simulink model "simulate"  (R2023a)
settings: Solver=VariableStepAuto  StartTime=0.0  StopTime=20  RelTol=1e-3
settings Model: Creator=dell  LastModifiedBy=zhs20
settings ModelReferenceCC: EnableRefExpFcnMdlSchedulingChecks=on

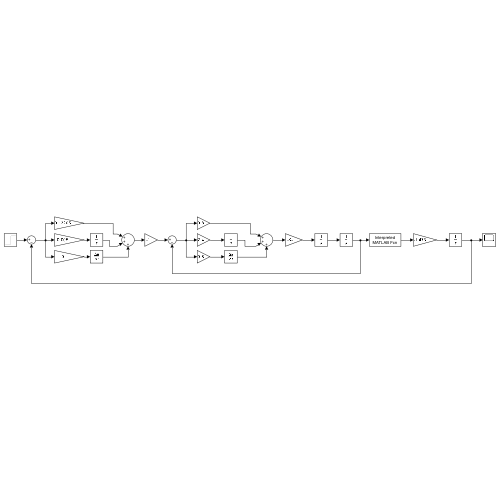
[thumbnail: Simulink's stored preview of the top-level diagram]
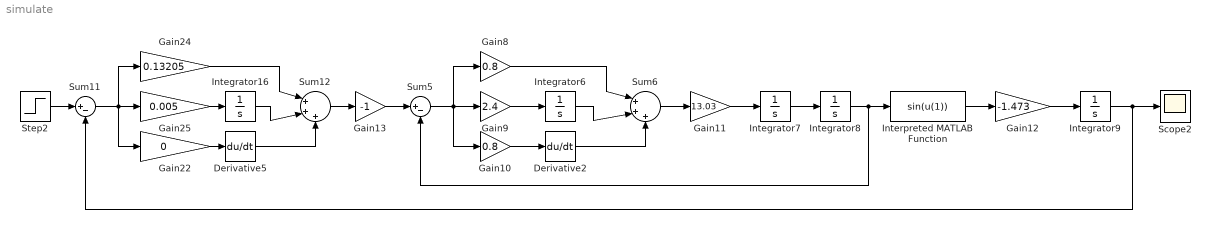
== system simulate ==
  Derivative2 : Derivative
  Derivative5 : Derivative
  Gain10 : Gain  Gain=0.8
  Gain11 : Gain  Gain=13.03
  Gain12 : Gain  Gain=-1.473
  Gain13 : Gain  Gain=-1
  Gain22 : Gain  Gain=0
  Gain24 : Gain  Gain=0.13205
  Gain25 : Gain  Gain=0.005
  Gain8 : Gain  Gain=0.8
  Gain9 : Gain  Gain=2.4
  Integrator{6..9,16} (5 alike) : Integrator
  Interpreted MATLAB Function : MATLABFcn  MATLABFcn=sin(u(1))
  Scope2 : Scope
  Step2 : Step  After=3.14  SampleTime=0
  Sum11 : Sum  Inputs=|+-
  Sum12 : Sum  Inputs=|+++
  Sum5 : Sum  Inputs=|+-
  Sum6 : Sum  Inputs=|+++
  wires:
  Integrator9/1 -> Scope2/1, Sum11/2
  Step2/1 -> Sum11/1
  Gain22/1 -> Derivative5/1
  Sum11/1 -> Gain24/1, Gain25/1, Gain22/1
  Integrator16/1 -> Sum12/2
  Derivative5/1 -> Sum12/3
  Gain12/1 -> Integrator9/1
  Integrator8/1 -> Interpreted MATLAB Function/1, Sum5/2
  Integrator7/1 -> Integrator8/1
  Gain24/1 -> Sum12/1
  Gain11/1 -> Integrator7/1
  Sum12/1 -> Gain13/1
  Gain25/1 -> Integrator16/1
  Gain9/1 -> Integrator6/1
  Derivative2/1 -> Sum6/3
  Gain10/1 -> Derivative2/1
  Interpreted MATLAB Function/1 -> Gain12/1
  Integrator6/1 -> Sum6/2
  Sum6/1 -> Gain11/1
  Gain13/1 -> Sum5/1
  Sum5/1 -> Gain8/1, Gain9/1, Gain10/1
  Gain8/1 -> Sum6/1
